simulink model "frenagem_suave"  (R2016a)
settings: Solver=ode45  StartTime=0.0  StopTime=40  FixedStep=.03  MinStep=.04  RelTol=1
libraries: dspvision x2, visionsources x1
settings Model: Creator=vmaraccini  LastModifiedBy=vmaraccini-personal
settings DataIOCC: LimitDataPoints=on  SaveFormat=Array
settings HardwareCC: ProdBitPerPointer=32  ProdLargestAtomicFloat=None  ProdIntDivRoundTo=Undefined  ProdEndianess=Unspecified  ProdWordSize=32  ProdHWDeviceType=32-bit Generic
settings ModelReferenceCC: PropagateSignalLabelsOutOfModel=off
settings ConfigComp: CovModelRefEnable=Off

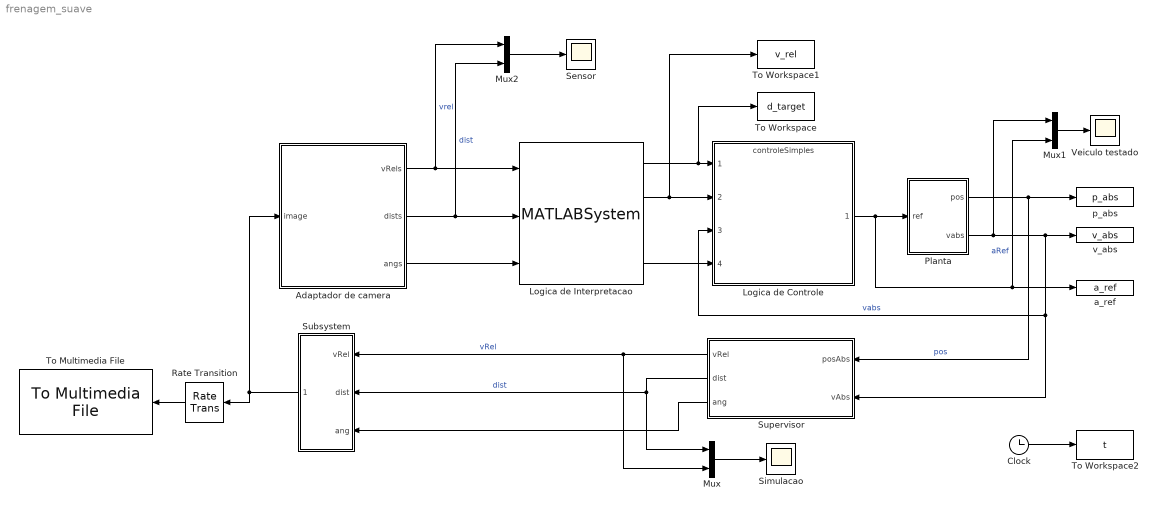
== system frenagem_suave ==
  Adaptador de camera : Subsystem
  Clock : Clock
  Logica de Controle : ModelReference  ModelNameDialog=controleSimples.slx  SimulationMode=Normal  ModelReferenceVersion=1.107
  Logica de Interpretacao : MATLABSystem  System=Interpretacao  SimulateUsing=Interpreted execution
      mask Type: Interpretacao
      mask Display:
      | disp('Interpretacao');
      | port_label('input',1,'vrels');
      | port_label('input',2,'dists');
      | port_label('input',3,'angs');
      | port_label('output',1,'dist');
      | port_label('output',2,'vrel');
      | port_label('output',3,'ang');
      | port_label('output',4,'vmax');
  Mux : Mux  Inputs=2
  Mux1 : Mux  Inputs=2
  Mux2 : Mux  Inputs=2
  Planta : Subsystem
  Rate Transition : RateTransition  OutPortSampleTime=.0416
  Sensor : Scope
  Simulacao : Scope
  Subsystem : Subsystem
  Supervisor : Subsystem
  To Multimedia File : dspvision/To Multimedia File  outputFilename=camera_sim.avi  streamSelection=Video only  videoCompressor=MJPEG Compressor  audioCompressor=None (uncompressed)  imagePorts=One multidimensional signal  fileType=AVI  audioDatatype=Determine from input data type  fourcc=RGB  videoQuality=75  mj2000CompFactor=10
  To Workspace : ToWorkspace  VariableName=d_target  SampleTime=-1
      settings: Save2DSignal=2-D array (concatenate along first dimension)
  To Workspace1 : ToWorkspace  VariableName=v_rel  SampleTime=-1
      settings: Save2DSignal=2-D array (concatenate along first dimension)
  To Workspace2 : ToWorkspace  VariableName=t  SampleTime=-1
      settings: Save2DSignal=2-D array (concatenate along first dimension)
  Veiculo testado : Scope
  a_ref : ToWorkspace  VariableName=a_ref  SampleTime=-1
      settings: Save2DSignal=2-D array (concatenate along first dimension)
  p_abs : ToWorkspace  VariableName=p_abs  SampleTime=-1
      settings: Save2DSignal=2-D array (concatenate along first dimension)
  v_abs : ToWorkspace  VariableName=v_abs  SampleTime=-1
      settings: Save2DSignal=2-D array (concatenate along first dimension)
  wires:
  Planta/2(vabs) -> Supervisor/2(vAbs), Logica de Controle/3, v_abs/1, Mux1/1  "vabs"
  Logica de Controle/1 -> Planta/1(ref), Mux1/2, a_ref/1  "aRef"
  Planta/1(pos) -> Supervisor/1(posAbs), p_abs/1  "pos"
  Logica de Interpretacao/1 -> To Workspace/1, Logica de Controle/1
  Supervisor/1(vRel) -> Mux/2, Subsystem/1(vRel)  "vRel"
  Supervisor/2(dist) -> Mux/1, Subsystem/2(dist)  "dist"
  Mux/1 -> Simulacao/1
  Mux1/1 -> Veiculo testado/1
  Logica de Interpretacao/4 -> Logica de Controle/4
  Logica de Interpretacao/2 -> Logica de Controle/2, To Workspace1/1
  Adaptador de camera/3(angs) -> Logica de Interpretacao/3
  Adaptador de camera/1(vRels) -> Mux2/1, Logica de Interpretacao/1  "vrel"
  Adaptador de camera/2(dists) -> Mux2/2, Logica de Interpretacao/2  "dist"
  Mux2/1 -> Sensor/1
  Clock/1 -> To Workspace2/1
  Rate Transition/1 -> To Multimedia File/1
  Subsystem/1(image) -> Adaptador de camera/1(image), Rate Transition/1
  Supervisor/3(ang) -> Subsystem/3(ang)

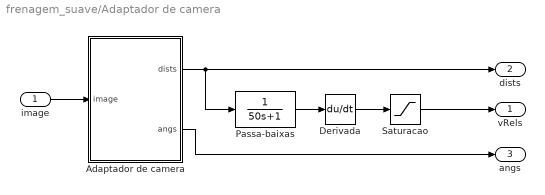
== system frenagem_suave/Adaptador de camera ==
  image : Inport
  Adaptador de camera : MATLAB Function  TreatAsAtomicUnit=on
  Derivada : Derivative
  Passa-baixas : TransferFcn  Numerator=1  Denominator=[50 1]
  Saturacao : Saturate  UpperLimit=100  LowerLimit=-10
  vRels : Outport
  dists : Outport  Port=2
  angs : Outport  Port=3
  wires:
  image/1 -> Adaptador de camera/1(image)
  Adaptador de camera/1(dists) -> Passa-baixas/1, dists/1
  Adaptador de camera/2(angs) -> angs/1
  Derivada/1 -> Saturacao/1
  Saturacao/1 -> vRels/1
  Passa-baixas/1 -> Derivada/1

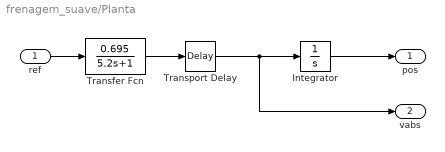
== system frenagem_suave/Planta ==
  ref : Inport
  Integrator : Integrator
  Transfer Fcn : TransferFcn  Numerator=[0 0.695]  Denominator=[5.2 1]
  Transport Delay : TransportDelay  DelayTime=0.5
  pos : Outport
  vabs : Outport  Port=2
  wires:
  Integrator/1 -> pos/1
  Transfer Fcn/1 -> Transport Delay/1
  ref/1 -> Transfer Fcn/1
  Transport Delay/1 -> vabs/1, Integrator/1

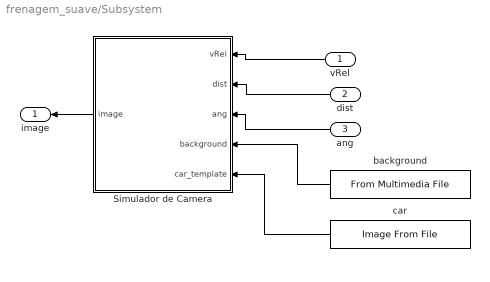
== system frenagem_suave/Subsystem ==
  vRel : Inport
  dist : Inport  Port=2
  ang : Inport  Port=3
  Simulador de Camera : MATLAB Function  TreatAsAtomicUnit=on
  background : dspvision/From Multimedia File  inputFilename=/Users/vmaraccini-personal/Documents/MATLAB/TCC/camera/camera_template.avi  loop=on  numPlays=inf  outputStreams=Video only  videoDataType=uint8  audioDataType=int16  inheritSampleTime=on  userDefinedSampleTime=1/30  noAudioOutput=off  isIntensityVideo=off  fourcc=Intensity  colorVideoFormat=One multidimensional signal  outputEOF=off  dataOrg=Column-major  audioFrameSize=1024  computeAudioFrameSize=off  outSamplingMode=Sample based
  car : visionsources/Image From File  Tag=vipblks_nd  FileName=/Users/vmaraccini-personal/Documents/MATLAB/TCC/camera/car_template.jpg  imagePorts=One multidimensional signal  Ts=inf  ImageDataType=uint8  Signed=on  WordLength=16  sdImageDataType=uint(8)  FractionLengthMode=User-defined  FractionLength=15  OutPortLabels=R|G|B
  image : Outport
  wires:
  ang/1 -> Simulador de Camera/3(ang)
  Simulador de Camera/1(image) -> image/1
  dist/1 -> Simulador de Camera/2(dist)
  vRel/1 -> Simulador de Camera/1(vRel)
  background/1 -> Simulador de Camera/4(background)
  car/1 -> Simulador de Camera/5(car_template)

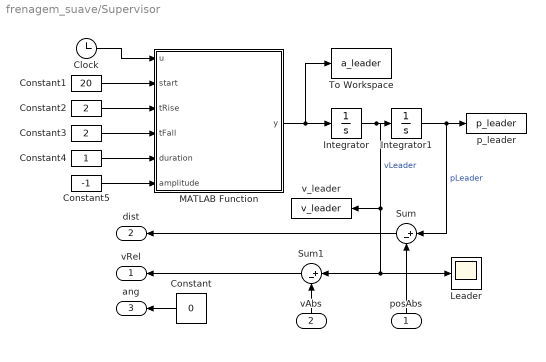
== system frenagem_suave/Supervisor ==
  posAbs : Inport
  vAbs : Inport  Port=2
  Clock : Clock
  Constant : Constant  Value=0
  Constant1 : Constant  Value=20
  Constant2 : Constant  Value=2
  Constant3 : Constant  Value=2
  Constant4 : Constant
  Constant5 : Constant  Value=-1
  Integrator : Integrator  InitialCondition=13.9
  Integrator1 : Integrator  InitialCondition=40
  Leader : Scope
  MATLAB Function : MATLAB Function  TreatAsAtomicUnit=on
  Sum : Sum  Inputs=|+-
  Sum1 : Sum  Inputs=|+-
  To Workspace : ToWorkspace  VariableName=a_leader  SampleTime=-1
      settings: Save2DSignal=2-D array (concatenate along first dimension)
  p_leader : ToWorkspace  VariableName=p_leader  SampleTime=-1
      settings: Save2DSignal=2-D array (concatenate along first dimension)
  v_leader : ToWorkspace  VariableName=v_leader  SampleTime=-1
      settings: Save2DSignal=2-D array (concatenate along first dimension)
  vRel : Outport
  dist : Outport  Port=2
  ang : Outport  Port=3
  wires:
  Integrator1/1 -> p_leader/1, Sum/1  "pLeader"
  Sum1/1 -> vRel/1
  vAbs/1 -> Sum1/2
  posAbs/1 -> Sum/2
  Sum/1 -> dist/1
  Integrator/1 -> v_leader/1, Leader/1, Sum1/1, Integrator1/1  "vLeader"
  Constant/1 -> ang/1
  MATLAB Function/1(y) -> To Workspace/1, Integrator/1
  Constant1/1 -> MATLAB Function/2(start)
  Constant2/1 -> MATLAB Function/3(tRise)
  Constant3/1 -> MATLAB Function/4(tFall)
  Constant4/1 -> MATLAB Function/5(duration)
  Constant5/1 -> MATLAB Function/6(amplitude)
  Clock/1 -> MATLAB Function/1(u)

== matlab function frenagem_suave/Subsystem/Simulador de Camera ==
  data: vRel input; image output; dist input; ang input; background input; car_template input
function image = simula_camera(vRel, dist, ang, background, car_template)
imgSize = 200;
dMax = 50;

image = uint8(zeros(imgSize, imgSize));

image = background;
% image = imresize(road_template, [imgSize, imgSize]);

% Adicionar ruido simulando fundo
image = image + uint8(255*rand(imgSize)/10); %10% de dMax

% Adicionar carro
if dist < 1
    dist = 1;
end
if dist > dMax
    dist = dMax;
end

% Adicionar ruido branco sobre o carro
tamanho = ceil(imgSize*.5*(1-dist/dMax));
tamanhoW = round(tamanho);
tamanhoH = round(0.7*tamanho);
displace = 15;

carro = rand(tamanhoH, tamanhoW)*0.1*(dist/dMax);
carro = carro + dist/dMax * ones(tamanhoH, tamanhoW);

image((end/2 - ceil(tamanhoH/2) + displace + 1) : (end/2 + floor(tamanhoH/2) + displace), ...
    (end/2 - ceil(tamanhoW/2) + 1) : end/2 + floor(tamanhoW/2)) = ...
    uint8(255*(1-carro));

end

== matlab function frenagem_suave/Supervisor/MATLAB Function ==
  data: u input; y output; start input; tRise input; tFall input; duration input; amplitude input
function y = aceleracao(u, start, tRise, tFall, duration, amplitude)
    y = (hv(u - start) - hv(u- (start+tRise) ))*amplitude.*((u-start)/tRise).^2 + ...
        (hv(u - (start+tRise)) - hv(u- (start+tRise+duration) ))*amplitude + ...
        (hv(u - (start+tRise+duration) ) - hv(u- (start+tRise+duration+tFall) ))*amplitude.*(1-((u- (start+tRise+duration) )/tFall).^2);
end

function y = hv(u)
    if u > 0
        y = 1;
    else
        y = 0;
    end
end

== matlab function frenagem_suave/Adaptador de camera/Adaptador de camera ==
  data: image input; dists output; angs output
function [dists, angs] = fcn(image)
numVehicles = 1;
dMax = 50;

dists = zeros(1,numVehicles);
angs = zeros(1,numVehicles);

dists = ones(1, numVehicles) * (1 - double(image(end/2,end/2))/255) * dMax;
angs = zeros(1, numVehicles);

end
